simulink model "blimp_simulation"  (R2021b)
settings: Solver=VariableStepAuto  StartTime=0.0  StopTime=200  RelTol=1e-3
values from neighbouring files (symbols this model uses):
  closed_loop = 1    [vars.mat]
  controller_on = 1    [vars.mat]
  Kd_a = 74    [vars.mat]
  Kd_f = -67.5    [vars.mat]
  Kd_h = -11    [vars.mat]
  Ki_a = 16    [vars.mat]
  Ki_f = 17    [vars.mat]
  Ki_h = 0.05    [vars.mat]
  Kp_a = 38    [vars.mat]
  Kp_f = 96    [vars.mat]
  Kp_h = 75    [vars.mat]
  N_a = 1.5    [vars.mat]
  N_f = 1.1    [vars.mat]
  N_h = 3.44    [vars.mat]
  opp_mode = 3    [blimp_setup.m]    (also in vars.mat = 2)
  slope = target_speed/radius    (= 0.0375)    [blimp_setup.m]    (also in vars.mat = 0)
  switch_freq = 5    [blimp_setup.m]    (also in vars.mat)
  switch_weight = 20    [blimp_setup.m]    (also in vars.mat = 75)
  target_alt = 0    [blimp_setup.m]    (also in vars.mat = 1)
  target_head = pi/2    (= 1.57079632679)    [blimp_setup.m]    (also in vars.mat)
  target_speed = 0.3    [blimp_setup.m]    (also in vars.mat)
undefined symbols (not defined in the file or in its folder): magnitude
libraries: slpidlib x3, cstblocks x3, simulink x1
settings Model: Creator=brend  LastModifiedBy=jcase

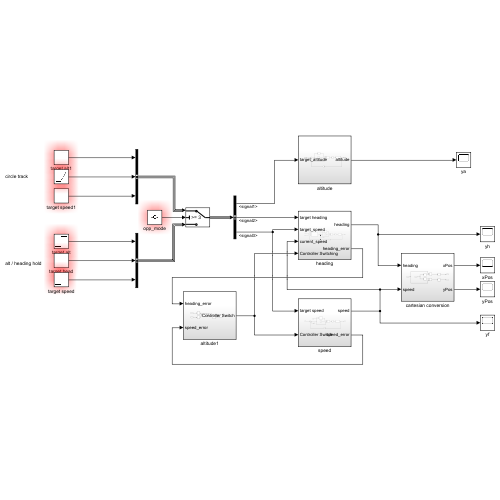
[thumbnail: Simulink's stored preview of the top-level diagram]
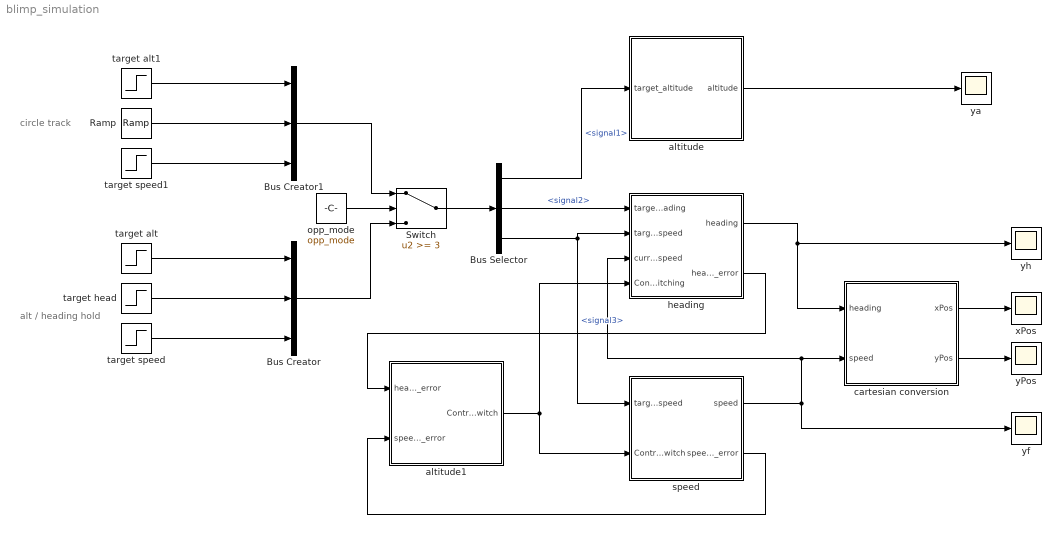
== system blimp_simulation ==
  note: alt / heading hold
  note: circle track
  Bus Creator : BusCreator  Inputs=3
  Bus Creator1 : BusCreator  Inputs=3
  Bus Selector : BusSelector  OutputSignals=signal1,signal2,signal3
  Ramp : simulink/Sources/Ramp  slope=slope  start=0  InitialOutput=0
  Switch : Switch  Threshold=3
  altitude : Subsystem
  altitude1 : Subsystem
  cartesian conversion : Subsystem
  heading : Subsystem
  opp_mode : Constant  Value=opp_mode
  speed : Subsystem
  target alt : Step  Time=0  After=target_alt  SampleTime=0
  target alt1 : Step  Time=0  After=target_alt  SampleTime=0
  target head : Step  Time=0  After=target_head  SampleTime=0
  target speed : Step  Time=0  After=target_speed  SampleTime=0
  target speed1 : Step  Time=0  After=target_speed  SampleTime=0
  xPos : Scope
  yPos : Scope
  ya : Scope
  yf : Scope
  yh : Scope
  wires:
  altitude/1(altitude) -> ya/1
  heading/1(heading) -> yh/1, cartesian conversion/1(heading)
  speed/1(speed) -> yf/1, heading/3(current_speed), cartesian conversion/2(speed)
  target alt/1 -> Bus Creator/1
  target head/1 -> Bus Creator/2
  target speed/1 -> Bus Creator/3
  target speed1/1 -> Bus Creator1/3
  target alt1/1 -> Bus Creator1/1
  opp_mode/1 -> Switch/2
  Switch/1 -> Bus Selector/1
  Bus Selector/1 -> altitude/1(target_altitude)  "<signal1>"
  Bus Selector/2 -> heading/1(target heading)  "<signal2>"
  Bus Selector/3 -> speed/1(target speed), heading/2(target_speed)  "<signal3>"
  Bus Creator1/1 -> Switch/1
  Bus Creator/1 -> Switch/3
  cartesian conversion/1(xPos) -> xPos/1
  cartesian conversion/2(yPos) -> yPos/1
  Ramp/1 -> Bus Creator1/2
  altitude1/1(Controller Switch) -> speed/2(Controller Switch), heading/4(Controller Switching)
  heading/2(heading_error) -> altitude1/1(heading_error)
  speed/2(speed_error) -> altitude1/2(speed_error)

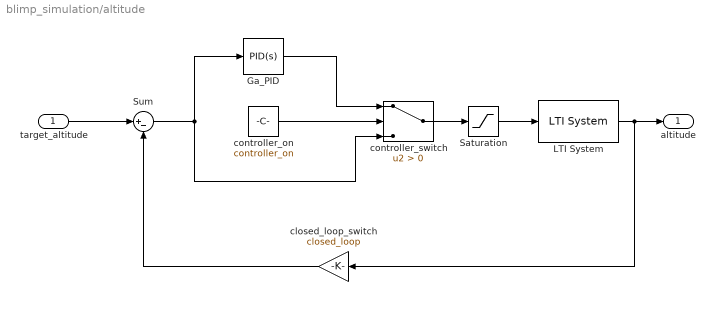
== system blimp_simulation/altitude ==
  target_altitude : Inport
  Ga_PID : slpidlib/PID Controller  Controller=PID  Form=Parallel  TimeDomain=Continuous-time  UseExternalTs=off  SampleTime=-1  IntegratorMethod=Forward Euler  FilterMethod=Forward Euler  ControllerParametersSource=internal  P=Kp_a  I=Ki_a  D=Kd_a  UseFilter=on  N=N_a  TunerSelectOption=Transfer Function Based (PID Tuner App)  InitialConditionSource=internal  InitialConditionForIntegrator=0  InitialConditionForFilter=0  DifferentiatorICPrevScaledInput=0  ExternalReset=none  TrackingMode=off  Kt=1  LimitOutput=off  SatLimitsSource=internal  UpperSaturationLimit=inf  LowerSaturationLimit=-inf  LinearizeAsGain=on  AntiWindupMode=none  Kb=1  POutMin=[]  POutMax=[]  IOutMin=[]  IOutMax=[]  DOutMin=[]  DOutMax=[]  NOutMin=[]  NOutMax=[]  SumOutMin=[]  SumOutMax=[]  SaturationOutMin=[]  SaturationOutMax=[]  PParamMin=[]  PParamMax=[]  IParamMin=[]  IParamMax=[]  DParamMin=[]  DParamMax=[]  NParamMin=[]  NParamMax=[]  KbParamMin=[]  KbParamMax=[]  KtParamMin=[]  KtParamMax=[]  KbOutMin=[]  KbOutMax=[]  KtOutMin=[]  KtOutMax=[]  IntegratorOutMin=[]  IntegratorOutMax=[]  FilterOutMin=[]  FilterOutMax=[]  SumI1OutMin=[]  SumI1OutMax=[]  SumI2OutMin=[]  SumI2OutMax=[]  SumI3OutMin=[]  SumI3OutMax=[]  SumI4OutMin=[]  SumI4OutMax=[]  SumDOutMin=[]  SumDOutMax=[]  DifferentiatorOutMin=[]  DifferentiatorOutMax=[]  FilterDiffOutCoefMin=[]  FilterDiffOutCoefMax=[]  ReciprocalOutMin=[]  ReciprocalOutMax=[]  SumDenOutMin=[]  SumDenOutMax=[]  SumNumOutMin=[]  SumNumOutMax=[]  DivideOutMin=[]  DivideOutMax=[]  UdiffTsProdOutMin=[]  UdiffTsProdOutMax=[]  NTsProdOutMin=[]  NTsProdOutMax=[]  UintegralTsProdOutMin=[]  UintegralTsProdOutMax=[]  UngainTsProdOutMin=[]  UngainTsProdOutMax=[]  IntegratorContinuousStateAttributes=''  IntegratorStateMustResolveToSignalObject=off  IntegratorRTWStateStorageClass=Auto  FilterContinuousStateAttributes=''  FilterStateMustResolveToSignalObject=off  FilterRTWStateStorageClass=Auto  ParallelPVariant=InternalParameters  IdealPVariant=Disabled  IVariant=InternalParameters  DVariant=InternalParameters  IntegratorVariant=Continuous  SatVariant=Disabled  AWVariant=Passthrough  PCopyVariant=Disabled  TRVariant=Disabled  FdbkBlocksVariant=Forward  IdealPFdbkVariant=Disabled  SatFdbkVariant=Disabled  DerivativeFilterVariant=ContFilter  NVariant=InternalParameters  NCopyVariant=Disabled  FilterICVariant=InternalICsFilter  IntegratorICVariant=InternalICs  ExternalResetVariant=Disabled  TRSumVariant=Passthrough  SumFdbkVariant=Disabled  SumVariant=Sum_PID  TsampFilterVariant=InternalTs  TsampNgainVariant=Passthrough  TsampIntegralVariant=Passthrough  ExternalSaturationOutDataTypeStr=Inherit: Same as second input
  LTI System : cstblocks/LTI System  sys=Ga  IC=[]
  Saturation : Saturate  UpperLimit=255  LowerLimit=0
  Sum : Sum  Inputs=|+-
  closed_loop_switch : Gain  Gain=closed_loop
  controller_on : Constant  Value=controller_on
  controller_switch : Switch  Criteria=u2 > Threshold
  altitude : Outport
  wires:
  target_altitude/1 -> Sum/1
  LTI System/1 -> closed_loop_switch/1, altitude/1
  controller_on/1 -> controller_switch/2
  Sum/1 -> Ga_PID/1, controller_switch/3
  closed_loop_switch/1 -> Sum/2
  Ga_PID/1 -> controller_switch/1
  controller_switch/1 -> Saturation/1
  Saturation/1 -> LTI System/1

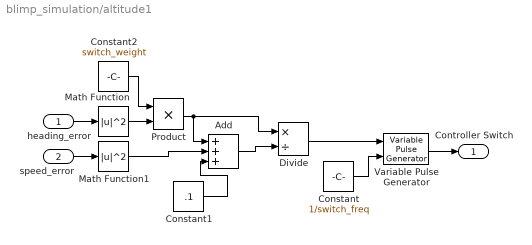
== system blimp_simulation/altitude1 ==
  heading_error : Inport
  speed_error : Inport  Port=2
  Add : Sum  Inputs=+++
  Constant : Constant  Value=1/switch_freq
  Constant1 : Constant  Value=.1
  Constant2 : Constant  Value=switch_weight
  Divide : Product  Inputs=*/
  Math Function : Math  Operator=magnitude^2  SaturateOnIntegerOverflow=on
  Math Function1 : Math  Operator=magnitude^2  SaturateOnIntegerOverflow=on
  Product : Product
  Variable Pulse Generator : VariablePulseGenerator  AllowZeroPulseWidth=on  SampleTime=0.1
  Controller Switch : Outport
  wires:
  Variable Pulse Generator/1 -> Controller Switch/1
  Constant/1 -> Variable Pulse Generator/2
  Add/1 -> Divide/2
  speed_error/1 -> Math Function1/1
  heading_error/1 -> Math Function/1
  Divide/1 -> Variable Pulse Generator/1
  Constant1/1 -> Add/3
  Math Function1/1 -> Add/2
  Product/1 -> Divide/1, Add/1
  Math Function/1 -> Product/2
  Constant2/1 -> Product/1

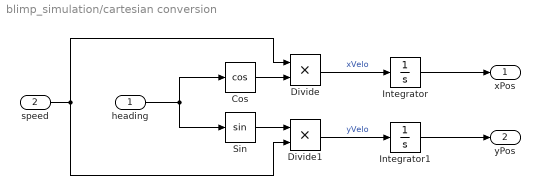
== system blimp_simulation/cartesian conversion ==
  heading : Inport
  speed : Inport  Port=2
  Cos : Trigonometry  Operator=cos
  Divide : Product  Inputs=**
  Divide1 : Product  Inputs=**
  Integrator : Integrator
  Integrator1 : Integrator
  Sin : Trigonometry
  xPos : Outport
  yPos : Outport  Port=2
  wires:
  heading/1 -> Cos/1, Sin/1
  speed/1 -> Divide1/2, Divide/1
  Cos/1 -> Divide/2
  Sin/1 -> Divide1/1
  Divide1/1 -> Integrator1/1  "yVelo"
  Divide/1 -> Integrator/1  "xVelo"
  Integrator/1 -> xPos/1
  Integrator1/1 -> yPos/1

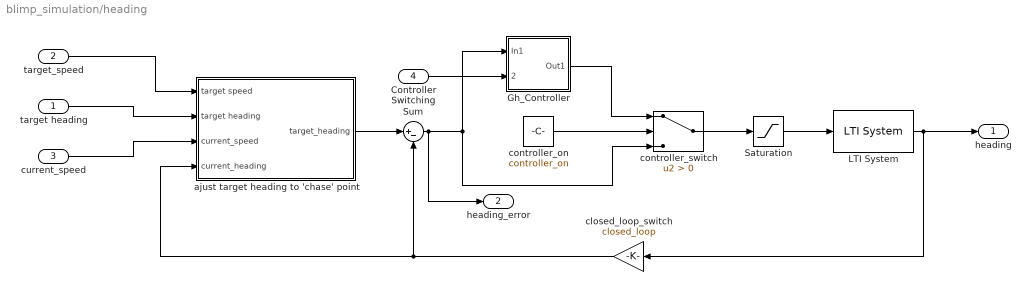
== system blimp_simulation/heading ==
  target heading : Inport
  target_speed : Inport  Port=2
  current_speed : Inport  Port=3
  Controller Switching : Inport  Port=4
  Gh_Controller : Subsystem
  LTI System : cstblocks/LTI System  sys=Gh  IC=[]
  Saturation : Saturate  UpperLimit=255  LowerLimit=-255
  Sum : Sum  Inputs=|+-
  ajust target heading to 'chase' point : Subsystem
  closed_loop_switch : Gain  Gain=closed_loop
  controller_on : Constant  Value=controller_on
  controller_switch : Switch  Criteria=u2 > Threshold
  heading : Outport
  heading_error : Outport  Port=2
  wires:
  closed_loop_switch/1 -> ajust target heading to 'chase' point/4(current_heading), Sum/2
  Sum/1 -> heading_error/1, Gh_Controller/1(In1), controller_switch/3
  controller_on/1 -> controller_switch/2
  LTI System/1 -> closed_loop_switch/1, heading/1
  Gh_Controller/1(Out1) -> controller_switch/1
  target heading/1 -> ajust target heading to 'chase' point/2(target heading)
  target_speed/1 -> ajust target heading to 'chase' point/1(target speed)
  current_speed/1 -> ajust target heading to 'chase' point/3(current_speed)
  ajust target heading to 'chase' point/1(target_heading) -> Sum/1
  Controller Switching/1 -> Gh_Controller/2(Controller Switching)
  controller_switch/1 -> Saturation/1
  Saturation/1 -> LTI System/1

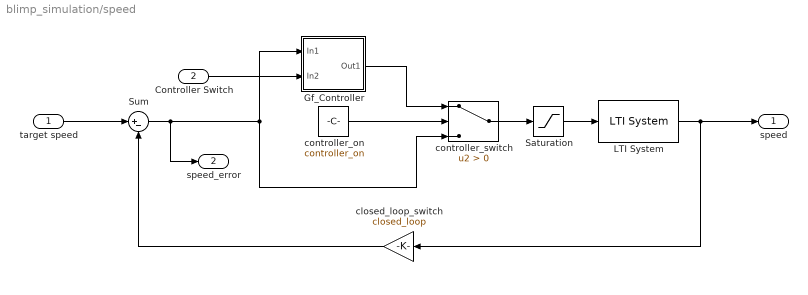
== system blimp_simulation/speed ==
  target speed : Inport
  Controller Switch : Inport  Port=2
  Gf_Controller : Subsystem
  LTI System : cstblocks/LTI System  sys=Gf  IC=[]
  Saturation : Saturate  UpperLimit=255  LowerLimit=0
  Sum : Sum  Inputs=|+-
  closed_loop_switch : Gain  Gain=closed_loop
  controller_on : Constant  Value=controller_on
  controller_switch : Switch  Criteria=u2 > Threshold
  speed : Outport
  speed_error : Outport  Port=2
  wires:
  closed_loop_switch/1 -> Sum/2
  Sum/1 -> speed_error/1, Gf_Controller/1(In1), controller_switch/3
  controller_on/1 -> controller_switch/2
  LTI System/1 -> closed_loop_switch/1, speed/1
  target speed/1 -> Sum/1
  Gf_Controller/1(Out1) -> controller_switch/1
  Controller Switch/1 -> Gf_Controller/2(In2)
  controller_switch/1 -> Saturation/1
  Saturation/1 -> LTI System/1

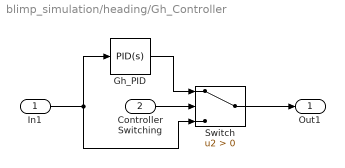
== system blimp_simulation/heading/Gh_Controller ==
  In1 : Inport
  Controller Switching : Inport  Port=2
  Gh_PID : slpidlib/PID Controller  Controller=PID  Form=Parallel  TimeDomain=Continuous-time  UseExternalTs=off  SampleTime=-1  IntegratorMethod=Forward Euler  FilterMethod=Forward Euler  ControllerParametersSource=internal  P=Kp_h  I=Ki_h  D=Kd_h  UseFilter=on  N=N_h  TunerSelectOption=Transfer Function Based (PID Tuner App)  InitialConditionSource=internal  InitialConditionForIntegrator=0  InitialConditionForFilter=0  DifferentiatorICPrevScaledInput=0  ExternalReset=none  TrackingMode=off  Kt=1  LimitOutput=off  SatLimitsSource=internal  UpperSaturationLimit=inf  LowerSaturationLimit=-inf  LinearizeAsGain=on  AntiWindupMode=none  Kb=1  POutMin=[]  POutMax=[]  IOutMin=[]  IOutMax=[]  DOutMin=[]  DOutMax=[]  NOutMin=[]  NOutMax=[]  SumOutMin=[]  SumOutMax=[]  SaturationOutMin=[]  SaturationOutMax=[]  PParamMin=[]  PParamMax=[]  IParamMin=[]  IParamMax=[]  DParamMin=[]  DParamMax=[]  NParamMin=[]  NParamMax=[]  KbParamMin=[]  KbParamMax=[]  KtParamMin=[]  KtParamMax=[]  KbOutMin=[]  KbOutMax=[]  KtOutMin=[]  KtOutMax=[]  IntegratorOutMin=[]  IntegratorOutMax=[]  FilterOutMin=[]  FilterOutMax=[]  SumI1OutMin=[]  SumI1OutMax=[]  SumI2OutMin=[]  SumI2OutMax=[]  SumI3OutMin=[]  SumI3OutMax=[]  SumI4OutMin=[]  SumI4OutMax=[]  SumDOutMin=[]  SumDOutMax=[]  DifferentiatorOutMin=[]  DifferentiatorOutMax=[]  FilterDiffOutCoefMin=[]  FilterDiffOutCoefMax=[]  ReciprocalOutMin=[]  ReciprocalOutMax=[]  SumDenOutMin=[]  SumDenOutMax=[]  SumNumOutMin=[]  SumNumOutMax=[]  DivideOutMin=[]  DivideOutMax=[]  UdiffTsProdOutMin=[]  UdiffTsProdOutMax=[]  NTsProdOutMin=[]  NTsProdOutMax=[]  UintegralTsProdOutMin=[]  UintegralTsProdOutMax=[]  UngainTsProdOutMin=[]  UngainTsProdOutMax=[]  IntegratorContinuousStateAttributes=''  IntegratorStateMustResolveToSignalObject=off  IntegratorRTWStateStorageClass=Auto  FilterContinuousStateAttributes=''  FilterStateMustResolveToSignalObject=off  FilterRTWStateStorageClass=Auto  ParallelPVariant=InternalParameters  IdealPVariant=Disabled  IVariant=InternalParameters  DVariant=InternalParameters  IntegratorVariant=Continuous  SatVariant=Disabled  AWVariant=Passthrough  PCopyVariant=Disabled  TRVariant=Disabled  FdbkBlocksVariant=Forward  IdealPFdbkVariant=Disabled  SatFdbkVariant=Disabled  DerivativeFilterVariant=ContFilter  NVariant=InternalParameters  NCopyVariant=Disabled  FilterICVariant=InternalICsFilter  IntegratorICVariant=InternalICs  ExternalResetVariant=Disabled  TRSumVariant=Passthrough  SumFdbkVariant=Disabled  SumVariant=Sum_PID  TsampFilterVariant=InternalTs  TsampNgainVariant=Passthrough  TsampIntegralVariant=Passthrough  ExternalSaturationOutDataTypeStr=Inherit: Same as second input
  Switch : Switch  Criteria=u2 > Threshold
  Out1 : Outport
  wires:
  In1/1 -> Gh_PID/1, Switch/3
  Gh_PID/1 -> Switch/1
  Switch/1 -> Out1/1
  Controller Switching/1 -> Switch/2

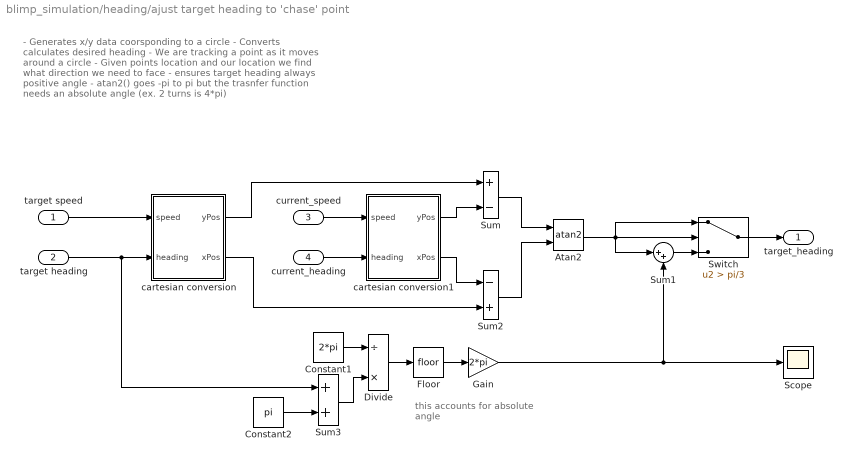
== system blimp_simulation/heading/ajust target heading to 'chase' point ==
  note: this accounts for
      | absolute angle
  note: - Generates x/y data coorsponding to a circle
      |
      | - Converts calculates desired heading
      | 	- We are tracking a point as it moves around a circle
      | 	- Given points location and our location we find what
      |  	  direction we need to face
      |
      | - ensures target heading always positive angle
      | 	- atan2() goes -pi to pi but the trasnfer function needs an
      |  	  absolute angle (ex. 2 turns is 4*pi)
  target speed : Inport
  target heading : Inport  Port=2
  current_speed : Inport  Port=3
  current_heading : Inport  Port=4
  Atan2 : Trigonometry  Operator=atan2
  Constant1 : Constant  Value=2*pi
  Constant2 : Constant  Value=pi
  Divide : Product  Inputs=/*
  Floor : Rounding
  Gain : Gain  Gain=2*pi
  Scope : Scope
  Sum : Sum  Inputs=+-
  Sum1 : Sum  Inputs=|++
  Sum2 : Sum  Inputs=-+
  Sum3 : Sum
  Switch : Switch  Criteria=u2 > Threshold  Threshold=pi/3
  cartesian conversion : Subsystem
  cartesian conversion1 : Subsystem
  target_heading : Outport
  wires:
  Sum/1 -> Atan2/1
  Sum2/1 -> Atan2/2
  Divide/1 -> Floor/1
  Floor/1 -> Gain/1
  Sum1/1 -> Switch/3
  Atan2/1 -> Sum1/1, Switch/2, Switch/1
  Constant1/1 -> Divide/1
  Sum3/1 -> Divide/2
  Gain/1 -> Scope/1, Sum1/2
  Constant2/1 -> Sum3/2
  target heading/1 -> Sum3/1, cartesian conversion/2(heading)
  target speed/1 -> cartesian conversion/1(speed)
  cartesian conversion/1(yPos) -> Sum/1
  cartesian conversion/2(xPos) -> Sum2/2
  current_heading/1 -> cartesian conversion1/2(heading)
  cartesian conversion1/1(yPos) -> Sum/2
  cartesian conversion1/2(xPos) -> Sum2/1
  current_speed/1 -> cartesian conversion1/1(speed)
  Switch/1 -> target_heading/1

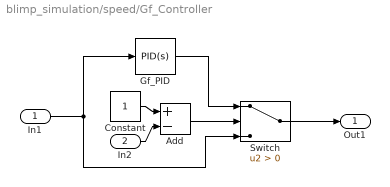
== system blimp_simulation/speed/Gf_Controller ==
  In1 : Inport
  In2 : Inport  Port=2
  Add : Sum  Inputs=+-
  Constant : Constant
  Gf_PID : slpidlib/PID Controller  Controller=PID  Form=Parallel  TimeDomain=Continuous-time  UseExternalTs=off  SampleTime=-1  IntegratorMethod=Forward Euler  FilterMethod=Forward Euler  ControllerParametersSource=internal  P=Kp_f  I=Ki_f  D=Kd_f  UseFilter=on  N=N_f  TunerSelectOption=Transfer Function Based (PID Tuner App)  InitialConditionSource=internal  InitialConditionForIntegrator=0  InitialConditionForFilter=0  DifferentiatorICPrevScaledInput=0  ExternalReset=none  TrackingMode=off  Kt=1  LimitOutput=off  SatLimitsSource=internal  UpperSaturationLimit=inf  LowerSaturationLimit=-inf  LinearizeAsGain=on  AntiWindupMode=none  Kb=1  POutMin=[]  POutMax=[]  IOutMin=[]  IOutMax=[]  DOutMin=[]  DOutMax=[]  NOutMin=[]  NOutMax=[]  SumOutMin=[]  SumOutMax=[]  SaturationOutMin=[]  SaturationOutMax=[]  PParamMin=[]  PParamMax=[]  IParamMin=[]  IParamMax=[]  DParamMin=[]  DParamMax=[]  NParamMin=[]  NParamMax=[]  KbParamMin=[]  KbParamMax=[]  KtParamMin=[]  KtParamMax=[]  KbOutMin=[]  KbOutMax=[]  KtOutMin=[]  KtOutMax=[]  IntegratorOutMin=[]  IntegratorOutMax=[]  FilterOutMin=[]  FilterOutMax=[]  SumI1OutMin=[]  SumI1OutMax=[]  SumI2OutMin=[]  SumI2OutMax=[]  SumI3OutMin=[]  SumI3OutMax=[]  SumI4OutMin=[]  SumI4OutMax=[]  SumDOutMin=[]  SumDOutMax=[]  DifferentiatorOutMin=[]  DifferentiatorOutMax=[]  FilterDiffOutCoefMin=[]  FilterDiffOutCoefMax=[]  ReciprocalOutMin=[]  ReciprocalOutMax=[]  SumDenOutMin=[]  SumDenOutMax=[]  SumNumOutMin=[]  SumNumOutMax=[]  DivideOutMin=[]  DivideOutMax=[]  UdiffTsProdOutMin=[]  UdiffTsProdOutMax=[]  NTsProdOutMin=[]  NTsProdOutMax=[]  UintegralTsProdOutMin=[]  UintegralTsProdOutMax=[]  UngainTsProdOutMin=[]  UngainTsProdOutMax=[]  IntegratorContinuousStateAttributes=''  IntegratorStateMustResolveToSignalObject=off  IntegratorRTWStateStorageClass=Auto  FilterContinuousStateAttributes=''  FilterStateMustResolveToSignalObject=off  FilterRTWStateStorageClass=Auto  ParallelPVariant=InternalParameters  IdealPVariant=Disabled  IVariant=InternalParameters  DVariant=InternalParameters  IntegratorVariant=Continuous  SatVariant=Disabled  AWVariant=Passthrough  PCopyVariant=Disabled  TRVariant=Disabled  FdbkBlocksVariant=Forward  IdealPFdbkVariant=Disabled  SatFdbkVariant=Disabled  DerivativeFilterVariant=ContFilter  NVariant=InternalParameters  NCopyVariant=Disabled  FilterICVariant=InternalICsFilter  IntegratorICVariant=InternalICs  ExternalResetVariant=Disabled  TRSumVariant=Passthrough  SumFdbkVariant=Disabled  SumVariant=Sum_PID  TsampFilterVariant=InternalTs  TsampNgainVariant=Passthrough  TsampIntegralVariant=Passthrough  ExternalSaturationOutDataTypeStr=Inherit: Same as second input
  Switch : Switch  Criteria=u2 > Threshold
  Out1 : Outport
  wires:
  In1/1 -> Switch/3, Gf_PID/1
  Add/1 -> Switch/2
  Gf_PID/1 -> Switch/1
  Switch/1 -> Out1/1
  Constant/1 -> Add/1
  In2/1 -> Add/2

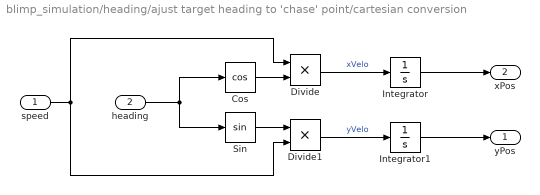
== system blimp_simulation/heading/ajust target heading to 'chase' point/cartesian conversion ==
  speed : Inport
  heading : Inport  Port=2
  Cos : Trigonometry  Operator=cos
  Divide : Product  Inputs=**
  Divide1 : Product  Inputs=**
  Integrator : Integrator
  Integrator1 : Integrator
  Sin : Trigonometry
  yPos : Outport
  xPos : Outport  Port=2
  wires:
  heading/1 -> Cos/1, Sin/1
  speed/1 -> Divide1/2, Divide/1
  Cos/1 -> Divide/2
  Sin/1 -> Divide1/1
  Divide1/1 -> Integrator1/1  "yVelo"
  Divide/1 -> Integrator/1  "xVelo"
  Integrator/1 -> xPos/1
  Integrator1/1 -> yPos/1

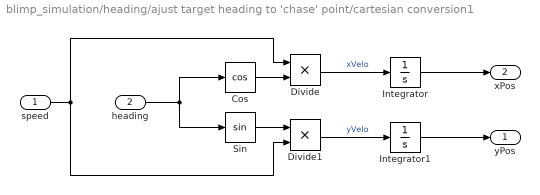
== system blimp_simulation/heading/ajust target heading to 'chase' point/cartesian conversion1 ==
  speed : Inport
  heading : Inport  Port=2
  Cos : Trigonometry  Operator=cos
  Divide : Product  Inputs=**
  Divide1 : Product  Inputs=**
  Integrator : Integrator
  Integrator1 : Integrator
  Sin : Trigonometry
  yPos : Outport
  xPos : Outport  Port=2
  wires:
  heading/1 -> Cos/1, Sin/1
  speed/1 -> Divide1/2, Divide/1
  Cos/1 -> Divide/2
  Sin/1 -> Divide1/1
  Divide1/1 -> Integrator1/1  "yVelo"
  Divide/1 -> Integrator/1  "xVelo"
  Integrator/1 -> xPos/1
  Integrator1/1 -> yPos/1
